simulink model "MA_Model"  (Simulink 7.3)
settings: Solver=FixedStepDiscrete  SolverMode=SingleTasking  StartTime=0.0  StopTime=878  FixedStep=1  RelTol=1e-3
PreLoadFcn:
  | [data,txt]=xlsread('BundDaily.xls');
  | Bund=data(:,end);
libraries: dspsrcs4 x1, dspsnks4 x1
settings Model: Creator=kassama  LastModifiedBy=kassama
settings OptimizationCC: InitFltsAndDblsToZero=on
settings DebuggingCC: SaveWithParameterizedLinksMsg=none
settings GRTTargetCC: TargetFcnLib=ansi_tfl_tmw.mat

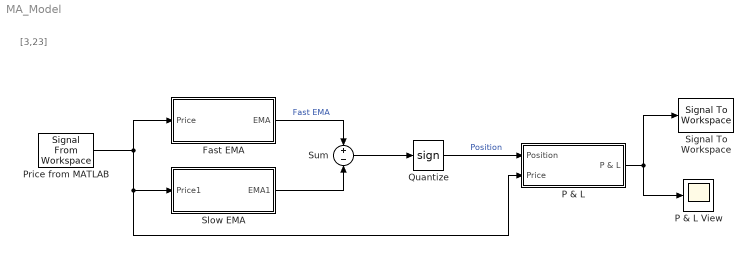
== system MA_Model ==
  note: [3,23]
  Fast EMA : Subsystem
  P & L : Subsystem
  P & L View : Scope
  Price from MATLAB : dspsrcs4/Signal From Workspace  SystemSampleTime=-1  X=Bund  Ts=1  nsamps=1  OutputAfterFinalValue=Setting to zero  ignoreOrWarnInputAndFrameLengths=off
  Quantize : Signum
  Signal To Workspace : dspsnks4/Signal To Workspace  SystemSampleTime=-1  VariableName=yout  FrameMode=Concatenate frames (2-D array)
      settings: FixptAsFi=off
  Slow EMA : Subsystem
  Sum : Sum  Inputs=+|-  OutDataType=sfix(16)  OutScaling=2^0
  wires:
  Slow EMA/1(EMA1) -> Sum/2
  Fast EMA/1(EMA) -> Sum/1  "Fast EMA"
  Price from MATLAB/1 -> Fast EMA/1(Price), Slow EMA/1(Price1), P & L/2(Price)
  Sum/1 -> Quantize/1
  Quantize/1 -> P & L/1(Position)  "Position"
  P & L/1(P & L) -> P & L View/1, Signal To Workspace/1

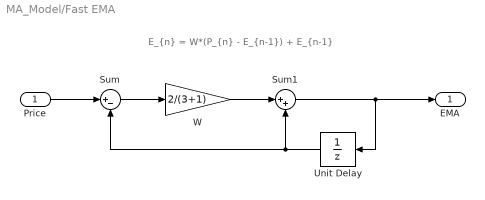
== system MA_Model/Fast EMA ==
  note: E_{n} = W*(P_{n} - E_{n-1}) + E_{n-1}
  Price : Inport  OutDataType=sfix(16)  OutScaling=2^0
  Sum : Sum  Inputs=|+-  OutDataType=sfix(16)  OutScaling=2^0
  Sum1 : Sum  Inputs=|++  OutDataType=sfix(16)  OutScaling=2^0
  Unit Delay : UnitDelay  X0=Bund(2)  SampleTime=-1
  W : Gain  Gain=2/(3+1)  ParameterDataType=sfix(16)  ParameterScaling=2^0  OutDataType=sfix(16)  OutScaling=2^0
  EMA : Outport  OutDataType=sfix(16)  OutScaling=2^0
  wires:
  Price/1 -> Sum/1
  Unit Delay/1 -> Sum/2, Sum1/2
  Sum/1 -> W/1
  W/1 -> Sum1/1
  Sum1/1 -> Unit Delay/1, EMA/1

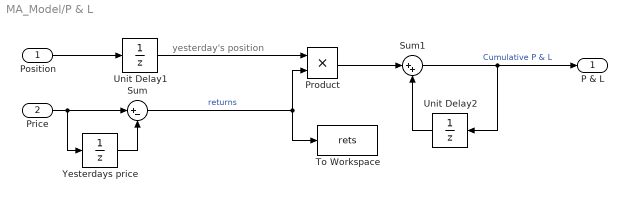
== system MA_Model/P & L ==
  note: yesterday's position
  Position : Inport  OutDataType=sfix(16)  OutScaling=2^0
  Price : Inport  Port=2  OutDataType=sfix(16)  OutScaling=2^0
  Product : Product  OutDataType=sfix(16)  OutScaling=2^0  RndMeth=Zero
  Sum : Sum  Inputs=|+-  OutDataType=sfix(16)  OutScaling=2^0
  Sum1 : Sum  Inputs=|++  OutDataType=sfix(16)  OutScaling=2^0
  To Workspace : ToWorkspace  VariableName=rets  SampleTime=-1  SaveFormat=Array
  Unit Delay1 : UnitDelay  SampleTime=-1
  Unit Delay2 : UnitDelay  SampleTime=-1
  Yesterdays price : UnitDelay  X0=Bund(2)  SampleTime=-1
  P & L : Outport  OutDataType=sfix(16)  OutScaling=2^0
  wires:
  Position/1 -> Unit Delay1/1
  Price/1 -> Sum/1, Yesterdays price/1
  Sum/1 -> Product/2, To Workspace/1  "returns"
  Unit Delay1/1 -> Product/1
  Product/1 -> Sum1/1
  Yesterdays price/1 -> Sum/2
  Unit Delay2/1 -> Sum1/2
  Sum1/1 -> P & L/1, Unit Delay2/1  "Cumulative P & L"

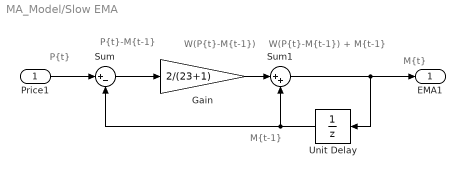
== system MA_Model/Slow EMA ==
  note: P{t}
  note: M{t}
  note: M{t-1}
  note: P{t}-M{t-1}
  note: W(P{t}-M{t-1})
  note: W(P{t}-M{t-1}) + M{t-1}
  Price1 : Inport  OutDataType=sfix(16)  OutScaling=2^0
  Gain : Gain  Gain=2/(23+1)  ParameterDataType=sfix(16)  ParameterScaling=2^0  OutDataType=sfix(16)  OutScaling=2^0
  Sum : Sum  Inputs=|+-  OutDataType=sfix(16)  OutScaling=2^0
  Sum1 : Sum  Inputs=|++  OutDataType=sfix(16)  OutScaling=2^0
  Unit Delay : UnitDelay  X0=Bund(2)
  EMA1 : Outport  OutDataType=sfix(16)  OutScaling=2^0
  wires:
  Price1/1 -> Sum/1
  Unit Delay/1 -> Sum/2, Sum1/2
  Sum/1 -> Gain/1
  Gain/1 -> Sum1/1
  Sum1/1 -> Unit Delay/1, EMA1/1
